simulink library "BUS_IN"  (R2018b)
settings: Solver=VariableStepAuto  StartTime=0.0  StopTime=10.0  RelTol=1e-3
settings Model: Creator=Alexander Koch  LastModifiedBy=ga69qig
settings SFSimCC: SimUseLocalCustomCode=off
settings RTWCC: RTWUseLocalCustomCode=off
settings CodeAppCC: StateflowObjectComments=on

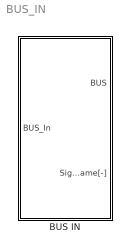
== system BUS_IN ==
  BUS IN : Subsystem
      mask help:
      | <Author> Alexander Koch, Benedikt Danquah based on Stefan Müller [1], Stephan Rohr [2]  </Author>
      |
      | <Date> 02/05/2017</Date>
      |
      | <Description>
      | Automated BUS IN Block for the Bus System. After the Bus In is connected and receives signals it is possible to choose the required signals by clicking on the block. After choosing the signals it is possible to push the Refresh button. This button builds the required amount of outputs, connects the Bus Selector and the Outputs and rename all the outputs with the corresponding signal name. The Block automaticlly disconnects the link to the library block after opening the first time
      | </Description>
      mask init:
      | BusInInitFct()
      settings: OpenFcn=|
      | set_param(gcb(),'LinkStatus','none')
      | open_system(gcb(),'mask')
      | open_system(strcat(gcb(),'/Bus Selector'),'Parameter')
      mask Help:
      | <Parameters>
      | -
      | </Parameters>
      | 
      | <Inputs>
      | Bus [Bus]
      | </Inputs>
      | 
      | <Outputs>
      | Bus [Bus]
      | SignalName[-]
      | </Outputs>
      | 
      | <Sources>
      | [1] S. Mueller, S. Rohr, W. Schmid, and M. Lienkamp, “Analysing the Influence of Driver Behaviour and Tuning Measures on Battery Aging and Residual Value of Electric Vehicles,” in Proc. EVS30 Symposium, Stuttgart, 2017, pp. 1–12.
      | [2] S. Rohr, “Technisch-wirtschaftliche Analyse des Zweitnutzungs- potentials von Lithium-Ionen-Traktionsbatterien,” Dissertation, Institute of Automotive Technology, Technical University Munich, Munich, 2018.
      | </Sources>
      mask DialogControl Container3 Prompt: Documentation:
      mask DialogControl Control3 Prompt: %<MaskHelp>
      mask DialogControl ParameterGroupVar Prompt: Refresh
      mask DialogControl RefreshOutputs Prompt: Refresh all Output Names
      mask DialogControl RefreshOutputs Callback: BusInInitFct()

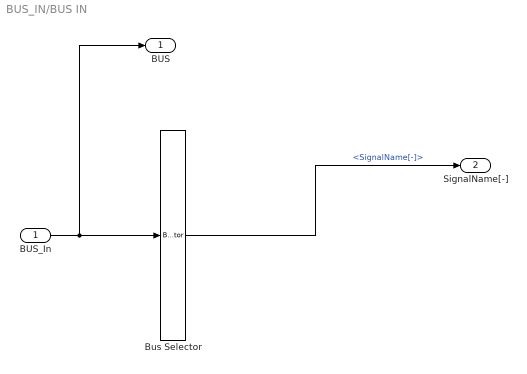
== system BUS_IN/BUS IN ==
  BUS_In : Inport
  Bus Selector : BusSelector  OutputSignals=Subsystem.SignalName[-]
  BUS : Outport
  SignalName[-] : Outport  Port=2
  wires:
  BUS_In/1 -> BUS/1, Bus Selector/1
  Bus Selector/1 -> SignalName[-]/1  "<SignalName[-]>"
